simulink model "PESO_ex2"  (R2020b)
settings: Solver=VariableStepAuto  StartTime=0.0  StopTime=10  FixedStep=1e-3  RelTol=1e-6
settings Model: Creator=Amir  LastModifiedBy=Amir
settings DataIOCC: ReturnWorkspaceOutputs=off

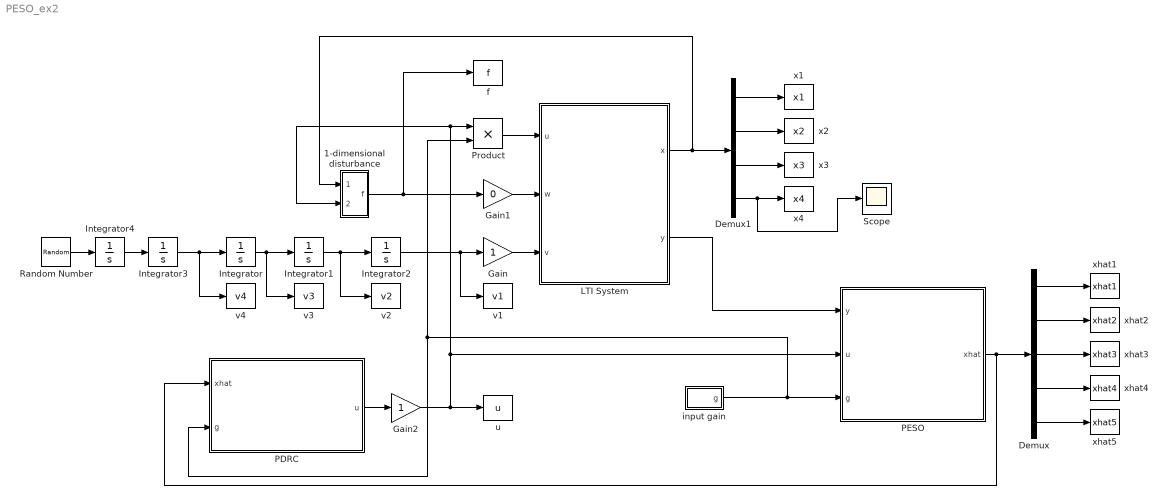
== system PESO_ex2 ==
  1-dimensional disturbance : Subsystem
  Demux : Demux  Outputs=5
  Demux1 : Demux
  Gain : Gain
  Gain1 : Gain  Gain=0
  Gain2 : Gain
  Integrator{,1..4} (5 alike) : Integrator
  LTI System : Subsystem  mask{n=4, m=1, k=1, A=[0 1 0 0;0 0 1 0;0 0 0 1;0 0 0 0], B=[0;0;0;1], C=[1 0 0 0], D=0, x0=[1;1;1;1]}
      mask prompts: n "Length of state vector (n):"; m "Length of input vector (m):"; k "Length of output vector (k):"; x0 "x(0):"
      mask DialogControl DescGroupVar Prompt: Main
      mask DialogControl DescTextVar Prompt: This block simulates a linear time-invariant (LTI) system. The system can be written as 'dx/dt=Ax+Bu+w' and 'y=Cx+Du+v'.
      mask DialogControl ParameterGroupVar Prompt: Dimensions
      mask DialogControl ParameterGroupVar_copy Prompt: Parameters
      mask DialogControl ParameterGroupVar_copy_copy Prompt: Initial Condition
  PDRC : Subsystem
  PESO : Subsystem  mask{n=4, tau=10, b=-[5;10;10;5;1], alpha=0.002, x0=10*[1;1;1;1], epsilon_t=1}
      mask prompts: n "Dimension of the system (n):"; tau "Convergence time (tau):"; b "Vector of observer gains (b):"; alpha "Mapping gain (alpha):"; x0 "Initial Estimated state (x0):"; epsilon_t "Switching tolerance (epsilon_t):"
      mask DialogControl DescGroupVar Prompt: Main
      mask DialogControl DescTextVar Prompt: Prescribed-time observer for unknown systems.
  Product : Product
  Random Number : RandomNumber  Variance=1e-6  SampleTime=1e-4
  Scope : Scope
  f : ToWorkspace  VariableName=f  SampleTime=-1
      settings: Save2DSignal=2-D array (concatenate along first dimension)
  input gain : Subsystem
  u : ToWorkspace  VariableName=u  SampleTime=-1
      settings: Save2DSignal=2-D array (concatenate along first dimension)
  v1 : ToWorkspace  VariableName=v1  SampleTime=-1
      settings: Save2DSignal=2-D array (concatenate along first dimension)
  v2 : ToWorkspace  VariableName=v2  SampleTime=-1
      settings: Save2DSignal=2-D array (concatenate along first dimension)
  v3 : ToWorkspace  VariableName=v3  SampleTime=-1
      settings: Save2DSignal=2-D array (concatenate along first dimension)
  v4 : ToWorkspace  VariableName=v4  SampleTime=-1
      settings: Save2DSignal=2-D array (concatenate along first dimension)
  x1 : ToWorkspace  VariableName=x1  SampleTime=-1
      settings: Save2DSignal=2-D array (concatenate along first dimension)
  x2 : ToWorkspace  VariableName=x2  SampleTime=-1
      settings: Save2DSignal=2-D array (concatenate along first dimension)
  x3 : ToWorkspace  VariableName=x3  SampleTime=-1
      settings: Save2DSignal=2-D array (concatenate along first dimension)
  x4 : ToWorkspace  VariableName=x4  SampleTime=-1
      settings: Save2DSignal=2-D array (concatenate along first dimension)
  xhat1 : ToWorkspace  VariableName=xhat1  SampleTime=-1
      settings: Save2DSignal=2-D array (concatenate along first dimension)
  xhat2 : ToWorkspace  VariableName=xhat2  SampleTime=-1
      settings: Save2DSignal=2-D array (concatenate along first dimension)
  xhat3 : ToWorkspace  VariableName=xhat3  SampleTime=-1
      settings: Save2DSignal=2-D array (concatenate along first dimension)
  xhat4 : ToWorkspace  VariableName=xhat4  SampleTime=-1
      settings: Save2DSignal=2-D array (concatenate along first dimension)
  xhat5 : ToWorkspace  VariableName=xhat5  SampleTime=-1
      settings: Save2DSignal=2-D array (concatenate along first dimension)
  wires:
  LTI System/2(y) -> PESO/1(y)
  PESO/1(xhat) -> Demux/1, PDRC/1(xhat)
  Demux/1 -> xhat1/1
  Demux/2 -> xhat2/1
  Demux/3 -> xhat3/1
  LTI System/1(x) -> 1-dimensional disturbance/1(x), Demux1/1
  Demux1/1 -> x1/1
  Demux1/2 -> x2/1
  1-dimensional disturbance/1(f) -> f/1, Gain1/1
  Demux/4 -> xhat4/1
  Demux/5 -> xhat5/1
  Demux1/3 -> x3/1
  Demux1/4 -> Scope/1, x4/1
  PDRC/1(u) -> Gain2/1
  input gain/1(g) -> Product/2, PDRC/2(g), PESO/3(g)
  Gain1/1 -> LTI System/2(w)
  Product/1 -> LTI System/1(u)
  Gain2/1 -> u/1, PESO/2(u), 1-dimensional disturbance/2(u), Product/1
  Integrator/1 -> v3/1, Integrator1/1
  Integrator1/1 -> Integrator2/1, v2/1
  Gain/1 -> LTI System/3(v)
  Integrator2/1 -> v1/1, Gain/1
  Random Number/1 -> Integrator4/1
  Integrator3/1 -> v4/1, Integrator/1
  Integrator4/1 -> Integrator3/1

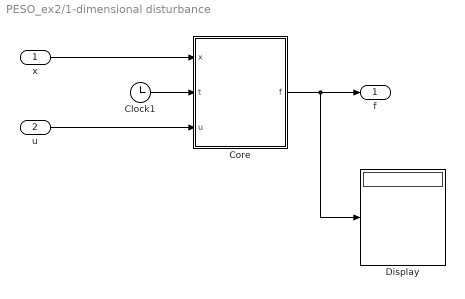
== system PESO_ex2/1-dimensional disturbance ==
  x : Inport
  u : Inport  Port=2
  Clock1 : Clock
  Core : MATLAB Function  TreatAsAtomicUnit=on
  Display : Display
  f : Outport
  wires:
  Core/1(f) -> Display/1, f/1
  Clock1/1 -> Core/2(t)
  x/1 -> Core/1(x)
  u/1 -> Core/3(u)

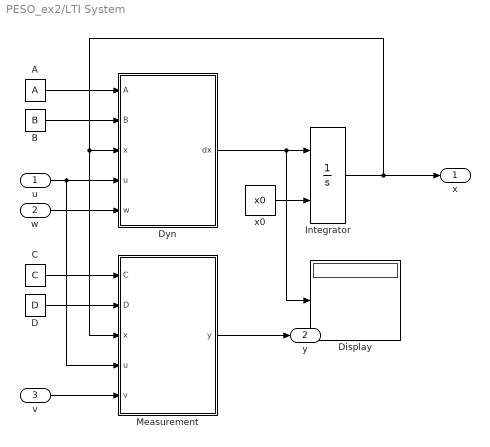
== system PESO_ex2/LTI System ==
  u : Inport
  w : Inport  Port=2
  v : Inport  Port=3
  A : Constant  Value=A
  B : Constant  Value=B
  C : Constant  Value=C
  D : Constant  Value=D
  Display : Display
  Dyn : MATLAB Function  TreatAsAtomicUnit=on
  Integrator : Integrator  InitialConditionSource=external
  Measurement : MATLAB Function  TreatAsAtomicUnit=on
  x0 : Constant  Value=x0
  x : Outport
  y : Outport  Port=2
  wires:
  v/1 -> Measurement/5(v)
  w/1 -> Dyn/5(w)
  u/1 -> Measurement/4(u), Dyn/4(u)
  Dyn/1(dx) -> Display/1, Integrator/1
  x0/1 -> Integrator/2
  B/1 -> Dyn/2(B)
  A/1 -> Dyn/1(A)
  C/1 -> Measurement/1(C)
  D/1 -> Measurement/2(D)
  Measurement/1(y) -> y/1
  Integrator/1 -> Measurement/3(x), Dyn/3(x), x/1

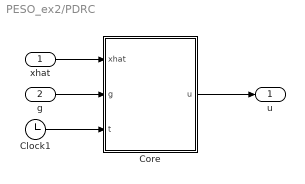
== system PESO_ex2/PDRC ==
  xhat : Inport
  g : Inport  Port=2
  Clock1 : Clock
  Core : MATLAB Function  TreatAsAtomicUnit=on
  u : Outport
  wires:
  Core/1(u) -> u/1
  Clock1/1 -> Core/3(t)
  xhat/1 -> Core/1(xhat)
  g/1 -> Core/2(g)

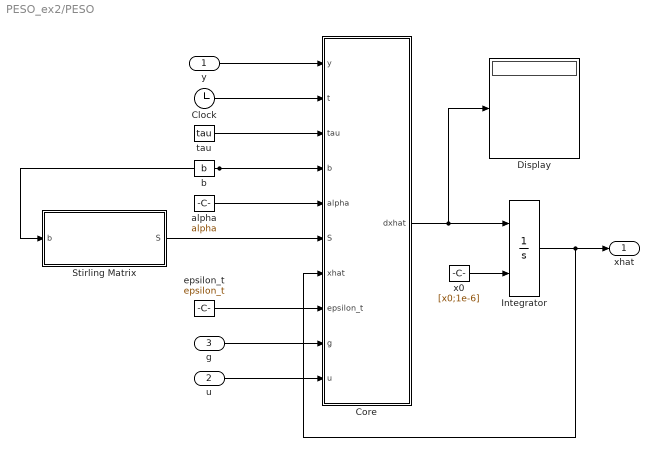
== system PESO_ex2/PESO ==
  y : Inport
  u : Inport  Port=2
  g : Inport  Port=3
  Clock : Clock
  Core : MATLAB Function  TreatAsAtomicUnit=on
  Display : Display
  Integrator : Integrator  InitialConditionSource=external
  Stirling Matrix : MATLAB Function  TreatAsAtomicUnit=on
  alpha : Constant  Value=alpha
  b : Constant  Value=b
  epsilon_t : Constant  Value=epsilon_t
  tau : Constant  Value=tau
  x0 : Constant  Value=[x0;1e-6]
  xhat : Outport
  wires:
  alpha/1 -> Core/5(alpha)
  b/1 -> Core/4(b), Stirling Matrix/1(b)
  y/1 -> Core/1(y)
  tau/1 -> Core/3(tau)
  Clock/1 -> Core/2(t)
  Stirling Matrix/1(S) -> Core/6(S)
  Core/1(dxhat) -> Display/1, Integrator/1
  x0/1 -> Integrator/2
  Integrator/1 -> xhat/1, Core/7(xhat)
  epsilon_t/1 -> Core/8(epsilon_t)
  u/1 -> Core/10(u)
  g/1 -> Core/9(g)

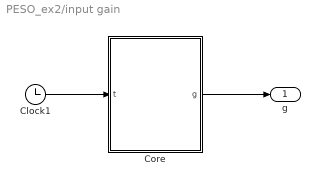
== system PESO_ex2/input gain ==
  Clock1 : Clock
  Core : MATLAB Function  TreatAsAtomicUnit=on
  g : Outport
  wires:
  Core/1(g) -> g/1
  Clock1/1 -> Core/1(t)

== matlab function PESO_ex2/LTI System/Measurement ==
  data: C input size=[k n]; D input size=[k m]; x input size=[n 1]; u input size=[m 1]; y output size=[k 1]; v input size=[k 1]
function y  = y_gen(C,D,x,u,v)

y = C*x+D*u+v;

== matlab function PESO_ex2/LTI System/Dyn ==
  data: A input size=[n n]; B input size=[n m]; x input size=[n 1]; u input size=[m 1]; dx output size=[n 1]; w input size=[n 1]
function dx  = dx_gen(A,B,x,u,w)

dx = A*x+B*u+w;

== matlab function PESO_ex2/1-dimensional disturbance/Core ==
  data: x input size=[4 1]; t input; u input; f output
function f = fcn(x,t,u)

f=zeros(length(x),1);

f(end)=cos(u)+sin(t^2)+norm(x)*exp(-norm(x))*u;

== matlab function PESO_ex2/PESO/Core ==
  data: y input size=[1 1]; dxhat output size=[n+1 1]; t input size=[1 1]; tau input size=[1 1]; b input size=[n+1 1]; alpha input size=[1 1]; S input size=[n+2 n+2]; xhat input size=[n+1,1]; epsilon_t input; g input; u input
function dxhat = PTC_gen(y,t,tau,b,alpha,S,xhat,epsilon_t,g,u)

if t>tau-epsilon_t
    
    t=tau-epsilon_t;
    
end

n=length(b)-1;

dxhat=zeros(n+1,1);

p=zeros(n+1,1);

for i=1:n+1
    
    sum=0;
    
    for j=i:n+1
        
        sum=sum+S(j,i)*(b(n-j+2))*(-1)^(j-i)/(alpha^(n-j+2)*(tau-t)^(n-i+2));
        
    end
    
    p(n-i+2)=-S(n+2,i)*(-1)^(n-i+2)/(tau-t)^(n-i+2)+sum;
    
end

for i=1:n-1
    
    dxhat(i)=xhat(i+1)+p(i)*(xhat(1)-y);
    
end

dxhat(n)=xhat(n+1)+p(n)*(xhat(1)-y)+g*u;

dxhat(n+1)=p(n+1)*(xhat(1)-y);

== matlab function PESO_ex2/PESO/Stirling Matrix ==
  data: b input size=[n+1 1]; S output size=[n+2 n+2]
function S = Stirling_gen(b)

n=length(b)+1;

S=zeros(n,n);

for i=1:n
    
    for j=1:n
        
        if i>=j
            
            m=0;

            for l=0:j-1
    
                sum=1/factorial(j-1)*(-1)^l*(factorial(j-1)/(factorial(l)*factorial(j-1-l)))*(j-1-l)^(i-1);
                
                m=m+sum;
                
            end
            
            S(i,j)=m;
            
        end
        
    end
    
end

== matlab function PESO_ex2/PDRC/Core ==
  data: xhat input size=[5 1]; g input; t input; u output
function u = fcn(xhat,g,t)

if t<0
    
    u=0;
    
else
    
    u=1/g*(-xhat(5)-[10000;4000;600;40]'*(xhat(1:4,1)-1*[sin(t);cos(t);-sin(t);-cos(t)]));

end

== matlab function PESO_ex2/input gain/Core ==
  data: t input; g output
function g = fcn(t)

g=exp(cos(t)+sin(t));
